simulink model "Analog"  (R2026b)
settings: Solver=VariableStepAuto  StopTime=80
undefined symbols (not defined in the file or in its folder): RF
libraries: simulink x1
settings Model: Creator=jacob  LastModifiedBy=jacob
settings SimscapeCC: SimscapeLogType=all  SimscapeNominalValues="[{\"value\":\"1\",\"unit\":\"A\"},{\"value\":\"1\",\"unit\":\"bar\"},{\"value\":\"1\",\"unit\":\"cm^2\"},{\"value\":\"1\",\"unit\":\"cm^3/s\"},{\"value\":\"1\",\"unit\":\"kJ/kg\"},{\"value\":\"1\",\"unit\":\"kW\"},{\"value\":\"1\",\"unit\":\"l\"},{\"value\":\"1\",\"unit\":\"N\"},{\"value\":\"1\",\"unit\":\"N*m\"},{\"value\":\"1\",\"unit\":\"V\"},{\"value\":\"0.001\",\"unit\":\"Wb\"}]"  SimscapeUseEnergyAccounting=off

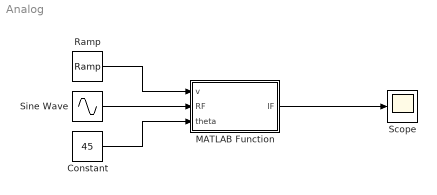
== system Analog ==
  Constant : Constant  Value=45
  MATLAB Function : MATLAB Function  TreatAsAtomicUnit=on
  Ramp : simulink/Sources/Ramp  slope=1  start=0  InitialOutput=0
  Scope : Scope
      settings: ActiveDisplayYMinimum=-697.85977286827347  ActiveDisplayYMaximum=8133.6593430707862
  Sine Wave : Sin  Frequency=2*pi*RF  SampleTime=0
  wires:
  Sine Wave/1 -> MATLAB Function/2(RF)
  MATLAB Function/1(IF) -> Scope/1
  Constant/1 -> MATLAB Function/3(theta)
  Ramp/1 -> MATLAB Function/1(v)

== matlab function Analog/MATLAB Function ==
  data: v input; IF output; RF input; theta input
function IF  = doppler(v, RF, theta)
%DOPPLER Summary of this function goes here
%   Detailed explanation goes here
arguments (Input)
    v
    RF
    theta
end

arguments (Output)
    IF
end

c = 299792458;
lambda = c/RF;
IF = (2*v/lambda)*cos(theta);
end
